simulink model "VehDyn14DOF"  (R2025a)
settings: Solver=VariableStepAuto  StartTime=0.0  StopTime=inf  FixedStep=0.001  RelTol=1e-3
model workspace (MAT data in the model file):
  ssEnable = Simulink.Parameter
  ssEnable.Value = 0
  ssEnable.Complexity = 'real'
  ssEnable.Dimensions = [1 1]
  ssEnable.DataType = 'boolean'
  xdot_r = Simulink.Parameter
  xdot_r.Value = 2.7778
  xdot_r.Complexity = 'real'
  xdot_r.Dimensions = [1 1]
  xdot_r.DataType = 'auto'
values from neighbouring files (symbols this model uses):
  AccPwrbp = 0.0 3.0779560993538198    [vehDyn14DOF.sldd]
  AccSpdbp = 256.49641719585139 641.24104298962845    [vehDyn14DOF.sldd]
  Downshift_Speeds = 9.5625 12.9375 16.3125 19.6875 23.0625 26.4375 29.8125 33.1875 36.5625 39.9375 43.3125 46.687499999999986 47.8125 51.187499999999986 54.562499999999986 57.9375 59.0625 62.4375 65.8125 69.1875 68.90625 72.84375 76.78125 80.71875 78.75 83.25 87.75 92.25    [vehDyn14DOF.sldd]
  EngRevLim = 7000.0    [vehDyn14DOF.sldd]
  F0z = 2886.0 2907.0    [vehDyn14DOF.sldd]
  Pedal_Positions = 0.1 0.4 0.5 0.9    [vehDyn14DOF.sldd]
  Trans = 0.01    [vehDyn14DOF.sldd]
  Upshift_Speeds = 12.9375 16.3125 19.6875 33.0 26.4375 29.8125 33.1875 52.5 39.9375 43.3125 46.687499999999986 77.25 51.187499999999986 54.562499999999986 57.9375 100.5 62.4375 65.8125 69.1875 138.75 72.84375 76.78125 80.71875 161.875 83.25 87.75 92.25 185.0    [vehDyn14DOF.sldd]
  VEH = 1575.0    [vehDyn14DOF.sldd]
undefined symbols (not defined in the file or in its folder): AccelCmd, CurvGradRef, CurvRef, DecelCmd, DiscIntNeverNeededParam, egoVehDyn, EnblAccelCmd, EnblDecelCmd, EnblSteerCmd, GearCmd, Gnd, Iz, lambda_mux, lambda_muy, lf, LngRef, lr, LtrRef, m, max_dc, maxSteer, PhiRef, SteerCmd, steeringGain, SteerZero, Wind, XRef, YRef, Z
libraries: simulink x14, autolibutils x13, autolibsharedcoupling x11, vehdynlibtire x10, vehdynlibsuspension x8, sharedtransform x5, autolibshareddiff x5, shared6dof x2, slpidlib x1, autolibtranscontrolscommon x1, vehdynlibdriver x1, autolibshared x1
(part 1 of 10)
CloseFcn:
  | Simulink.data.dictionary.closeAll('vehDyn14DOF.sldd', '-discard')
settings Model: DataDictionary=vehDyn14DOF.sldd  Creator=The MathWorks, Inc.  LastModifiedBy=sdussani
settings SolverCC: MaxZcPerStep=1.0
settings DataIOCC: InitialState=refModelOP  SignalLogging=off
settings OptimizationCC: ReuseModelBlockBuffer=off  ZeroExternalMemoryAtStartup=off  ZeroInternalMemoryAtStartup=off
settings DebuggingCC: UnconnectedInputMsg=warning  UnconnectedOutputMsg=warning  UnconnectedLineMsg=warning  SubsystemReferenceDiagnosticForUnitTest=warning
settings ModelReferenceCC: EnableRefExpFcnMdlSchedulingChecks=on
settings RTWCC: GenerateReport=on  LaunchReport=on  TargetLang=C++  GPUComputeCapability=3.5  DLArmComputeVersion=19.05
settings GRTTargetCC: TargetLangStandard=C++03 (ISO)  MatFileLogging=off  CodeInterfacePackaging=C++ class

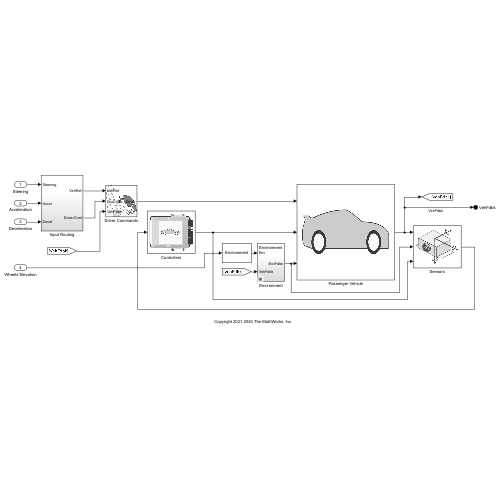
[thumbnail: Simulink's stored preview of the top-level diagram]
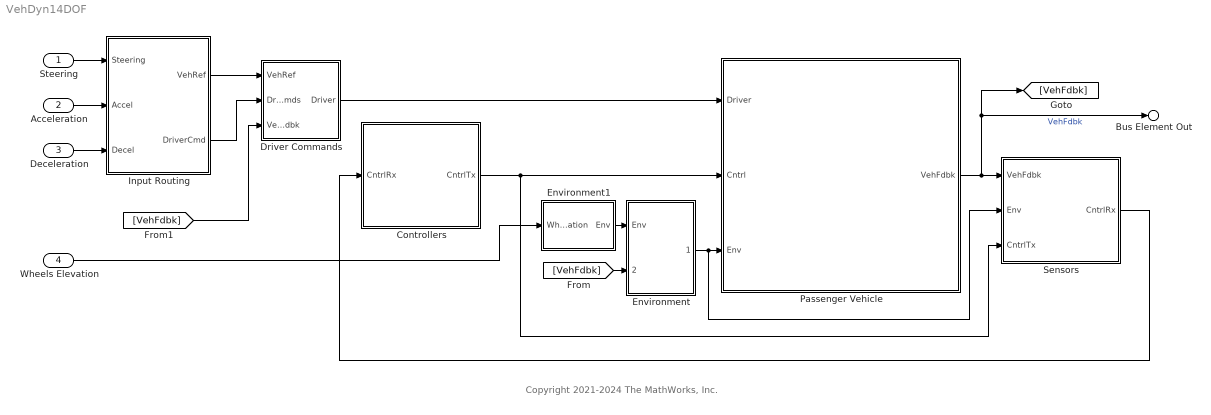
== system VehDyn14DOF ==
  note: Copyright 2021-2024 The MathWorks, Inc.
  Steering : Inport
  Acceleration : Inport  Port=2
  Deceleration : Inport  Port=3
  Wheels Elevation : Inport  Port=4
  Controllers : Subsystem
      mask Display: image('$imagefile'); % Use "Edit Image" on toolstrip to change.
  Driver Commands : Subsystem  VariantControl=0
      mask Display: image('driverlatlong.png');
  Environment : Subsystem  Variant=on  VariantControlMode=label  VariantControl=Choice  LabelModeActiveChoice=Choice
  Environment1 : Subsystem
      mask Display: disp('Environment')
  Input Routing : Subsystem  VariantControl=0
  Passenger Vehicle : Subsystem
      mask Display: image('$imagefile'); % Use "Edit Image" on toolstrip to change.
  Sensors : Subsystem
      mask Display: image('sensorimu.png'); % Use "Edit Image" on toolstrip to change.
  Bus Element Out : Outport  PortName=VehFdbk
  wires:
  Passenger Vehicle/1(VehFdbk) -> Bus Element Out/1, [VehFdbk], Sensors/1(VehFdbk)  "VehFdbk"
  Sensors/1(CntrlRx) -> Controllers/1(CntrlRx)
  Controllers/1(CntrlTx) -> Passenger Vehicle/2(Cntrl), Sensors/3(CntrlTx)
  Driver Commands/1(Driver) -> Passenger Vehicle/1(Driver)
  Input Routing/1(VehRef) -> Driver Commands/1(VehRef)
  Input Routing/2(DriverCmd) -> Driver Commands/2(DrvCmds)
  Environment1/1(Env) -> Environment/1(Env)
  [VehFdbk] -> Environment/2(VehFdbk)
  Environment/1(EnvFdbk) -> Sensors/2(Env), Passenger Vehicle/3(Env)
  [VehFdbk] -> Driver Commands/3(VehFdbk)
  Acceleration/1 -> Input Routing/2(Accel)
  Steering/1 -> Input Routing/1(Steering)
  Deceleration/1 -> Input Routing/3(Decel)
  Wheels Elevation/1 -> Environment1/1(Wheels Elevation)

== system VehDyn14DOF/Controllers ==
  CntrlRx : Inport
  Active Differential Control : Subsystem  Variant=on  VariantControlMode=label  LabelModeActiveChoice=0
  Brake Pressure Control : Subsystem  Variant=on  VariantControlMode=label  LabelModeActiveChoice=0
  Bus Creator : BusCreator  Inputs=1
  Bus Creator1 : BusCreator  Inputs=1
  Bus Creator2 : BusCreator  Inputs=2
  Bus Creator3 : BusCreator  Inputs=4
  Bus Creator4 : BusCreator  Inputs=1
  Bus Selector : BusSelector  OutputSignals=Driver.DecelFdbk,Wheels.Omega,IMU.Acc
  Bus Selector1 : BusSelector  OutputSignals=Driver.AccFdbk,Driver.DecelFdbk,Driver.GearFdbk,Engine.EngSpd,Wheels.Omega
  Bus Selector2 : BusSelector  OutputSignals=Driver.AccFdbk,Engine.EngSpd
  Bus Selector3 : BusSelector  OutputSignals=Driver.AccFdbk,Driver.DecelFdbk,Driver.SteerFdbk,Driver.GearFdbk,Wheels.Omega,IMU.Acc,IMU.pqr
  ECU : Subsystem  SystemSampleTime=.01
  Ground : Ground
  Transmission Controller : Subsystem  Variant=on  VariantControlMode=label  VariantControl=Variant1  LabelModeActiveChoice=3
  CntrlTx : Outport  VectorParamsAs1DForOutWhenUnconnected=off
  wires:
  Bus Selector2/1 -> ECU/2(<Accel>)  "<AccFdbk>"
  Bus Creator/1 -> Bus Creator3/1  "ECU"
  Bus Creator1/1 -> Bus Creator3/2  "Transmission"
  Bus Creator3/1 -> CntrlTx/1  "CntrlTx"
  Bus Creator4/1 -> Bus Creator3/4  "Diff"
  Active Differential Control/1(DiffPrsCmd) -> Bus Creator4/1  "DiffPrsCmd"
  Active Differential Control/2(TrqCmd) -> [DiffTrqCmd]
  ECU/1(EngTrqCmd) -> Bus Creator/1  "EngTrqCmd"
  Transmission Controller/1(" Gear") -> Bus Creator1/1  "GearCmd"
  [DiffTrqCmd] -> ECU/1(DiffTrqCmd)  "DiffTrqCmd"
  Ground/1 -> Transmission Controller/7(UpReq), Transmission Controller/8(DownReq)
  Bus Selector2/2 -> ECU/3(EngSpd)  "<EngSpd>"
  Bus Selector1/5 -> Transmission Controller/5(Omega)  "<Omega>"
  Bus Selector1/2 -> Transmission Controller/2(BrkCmd)  "<DecelFdbk>"
  Bus Selector1/3 -> Transmission Controller/3(GearReq)  "<GearFdbk>"
  Bus Selector1/4 -> Transmission Controller/4(EngSpd)  "<EngSpd>"
  Bus Selector1/1 -> Transmission Controller/1(Accel)  "<AccFdbk>"
  Bus Selector3/1 -> Active Differential Control/1(Accel)  "<AccFdbk>"
  Bus Selector3/2 -> Active Differential Control/2(BrkCmd)  "<DecelFdbk>"
  Bus Selector3/3 -> Active Differential Control/3(Steer)  "<SteerFdbk>"
  Bus Selector3/4 -> Active Differential Control/4(GearFdbk)  "<GearFdbk>"
  Bus Selector3/5 -> Active Differential Control/5(Omega)  "<Omega>"
  Bus Selector3/6 -> Active Differential Control/6(axayaz)  "<Acc>"
  Bus Selector3/7 -> Active Differential Control/7(pqr)  "<pqr>"
  Bus Selector/1 -> Brake Pressure Control/1(DecelFdbk)  "<DecelFdbk>"
  CntrlRx/1 -> Bus Selector/1, Bus Selector3/1, Bus Selector1/1, Bus Selector2/1
  Bus Selector/2 -> Brake Pressure Control/2(Omega)  "<Omega>"
  Bus Selector/3 -> Brake Pressure Control/3(Accel)  "<Acc>"
  Brake Pressure Control/1(BrkPrsCmd) -> Bus Creator2/1  "BrkPrsCmd"
  Bus Creator2/1 -> Bus Creator3/3  "Brake"
  Brake Pressure Control/2(ABSFlag) -> Bus Creator2/2, [ABSFlag]  "ABSFlag"
  [ABSFlag] -> Transmission Controller/6(ABSFlag)
  [ABSFlag] -> ECU/4(ABSFlag)

== system VehDyn14DOF/Driver Commands ==
  VehRef : Inport  OutDataTypeStr=Bus: BusVehRef
  DrvCmds : Inport  Port=2  OutDataTypeStr=Bus: BusDrvCmds
  VehFdbk : Inport  Port=3
  Bus Creator1 : BusCreator  Inputs=5
  Bus Selector : BusSelector  OutputSignals=Body.BdyFrm.Cg.Vel.xdot,Body.InertFrm.Geom.Disp.X,Body.InertFrm.Geom.Disp.Y,Body.InertFrm.Cg.Ang.psi,Body.BdyFrm.Cg.AngVel.r
  Bus Selector1 : BusSelector  OutputSignals=EnblSteerCmd,SteerCmd,SteerHld,SteerZero,EnblAccelCmd,AccelCmd,AccelHld,AccelZero,EnblDecelCmd,DecelCmd,DecelHld,DecelZero
  Bus Selector2 : BusSelector  OutputSignals=LngRef,XRef,YRef,PhiRef,CurvRef
  Dead Zone : DeadZone  LowerValue=-.5  UpperValue=.5  ZeroCross=off
  Gain : Gain  Gain=18*maxSteer
  Ground : Ground
  Ground1 : Ground
  Linear Predictive Driver : vehdynlibdriver/Predictive Driver  extAccelOvr=on  extDecelOvr=on  extAccelHld=on  extDecelHld=on  extAccelZero=on  extDecelZero=on  extSteerOvr=on  extSteerHld=on  extSteerZero=on  cntrlType=Predictive  cntrlTypeLat=Stanley  shftType=Reverse, Neutral, Drive  coordMode=SAE J670 (Z-down)  refType=Reference pose  velUnits=m/s  angUnits=rad  gearOut=on  steerOut=on  Kp=3  Ki=1  Kff=1  Kg=0  VehVelVec=[0 100]  KffVec=[.1 .1]  KpVec=[10 10]  KiVec=[5 5]  KgVec=[0 0]  vnom=5  Kaw=1  tauerr=.075  tau=.15  L=6  Kpt=20000  aR=200  bR=2.5  cR=.5  g=9.81  vecPose=off  dynamMode=on  PositionGainF=2.5  PositionGainR=2.5  YawRateGain=.2  DelayGain=.2  enableDrift=off  BetaRef=20*pi/180  KpBeta=1  KpDrift=2  KdDrift=1  KpPsi=6  KOmega=30  tOmega=1  a=VEH.FrontAxlePositionfromCG  b=VEH.RearAxlePositionfromCG  m=VEH.Mass  Cy_f=5000  Cy_r=7000  I=VEH.YawMomentInertia  Ksteer=18  theta=40*pi/180  Idl=1  Re=.3  lambda_mu=1  GearInit=1  tShift=.1  pdlVec=[0.1 0.4 0.5 0.9]  upShftTbl=[-1 12.9375 26.4375 39.9375 51.18749999999999 62.4375 72.84375 83.25;-1 16.3125 29.8125 43.3125 54.5624 65.8125 76.78125 87.75;-1 19.6875 33.1875 46.68749999999999 57.9375 69.1875 80.71875 92.25;-1 33 52.5 77.25 100.5 138.75 161.875 185]  dwnShftTbl=[-1 12.9375 26.4375 39.9375 51.18749999999999 62.4375 72.84375 83.25;-1 16.3125 29.8125 43.3125 54.5624 65.8125 76.78125 87.75;-1 19.6875 33.1875 46.68749999999999 57.9375 69.1875 80.71875 92.25;-1 33 52.5 77.25 100.5 138.75 161.875 185]  tClutch=.5  tRev=.5  tPark=120  UpGearVec="[0  1  2  3  4  5  6  7]"  DownGearVec="[1  2  3  4  5  6  7  8]"  aMode=2
  Mux : Mux  Inputs=3
  Steady State : Subsystem  VariantControl=Choice
  Terminator : Terminator
  Driver : Outport  VectorParamsAs1DForOutWhenUnconnected=off
  wires:
  Bus Creator1/1 -> Driver/1
  Bus Selector2/1 -> Linear Predictive Driver/1  "<LngRef>"
  VehFdbk/1 -> Bus Selector/1
  Bus Selector/2 -> Linear Predictive Driver/20  "<X>"
  Linear Predictive Driver/4 -> Bus Creator1/3  "decel_cmd"
  Linear Predictive Driver/2 -> Bus Creator1/1  "steer_cmd"
  Ground/1 -> Linear Predictive Driver/17
  Linear Predictive Driver/1 -> Terminator/1
  Linear Predictive Driver/3 -> Bus Creator1/2  "accel_cmd"
  Bus Selector/4 -> Linear Predictive Driver/22  "<psi>"
  Bus Selector/5 -> Linear Predictive Driver/23  "<r>"
  Bus Selector/1 -> Dead Zone/1  "<xdot>"
  Linear Predictive Driver/5 -> Bus Creator1/4  "gear_cmd"
  Bus Selector/3 -> Linear Predictive Driver/21  "<Y>"
  Dead Zone/1 -> Linear Predictive Driver/19
  Ground1/1 -> Mux/3
  Mux/1 -> Bus Creator1/5  "Ref"
  DrvCmds/1 -> Steady State/2(DrvCmds)
  Bus Selector1/1 -> Linear Predictive Driver/5  "<EnblSteerCmd>"
  Bus Selector1/2 -> Gain/1  "<SteerCmd>"
  Bus Selector1/3 -> Linear Predictive Driver/7  "<SteerHld>"
  Bus Selector1/4 -> Linear Predictive Driver/8  "<SteerZero>"
  Bus Selector1/5 -> Linear Predictive Driver/9  "<EnblAccelCmd>"
  Bus Selector1/6 -> Linear Predictive Driver/10  "<AccelCmd>"
  Bus Selector1/7 -> Linear Predictive Driver/11  "<AccelHld>"
  Bus Selector1/8 -> Linear Predictive Driver/12  "<AccelZero>"
  Bus Selector1/9 -> Linear Predictive Driver/13  "<EnblDecelCmd>"
  Bus Selector1/10 -> Linear Predictive Driver/14  "<DecelCmd>"
  Bus Selector1/11 -> Linear Predictive Driver/15  "<DecelHld>"
  Bus Selector1/12 -> Linear Predictive Driver/16  "<DecelZero>"
  VehRef/1 -> Steady State/1(VehRef)
  Bus Selector2/2 -> Mux/1, Linear Predictive Driver/2  "<XRef>"
  Bus Selector2/3 -> Mux/2, Linear Predictive Driver/3  "<YRef>"
  Bus Selector2/4 -> Linear Predictive Driver/4  "<PhiRef>"
  Bus Selector2/5 -> Linear Predictive Driver/18  "<CurvRef>"
  Steady State/1(Ref) -> Bus Selector2/1
  Steady State/2(Cmds) -> Bus Selector1/1
  Gain/1 -> Linear Predictive Driver/6

== system VehDyn14DOF/Environment ==
  Env : Inport
  VehFdbk : Inport  Port=2
  Environment : Subsystem  VariantControl=Choice
  EnvFdbk : Outport

== system VehDyn14DOF/Environment1 ==
  Wheels Elevation : Inport
  Bus Assignment : BusAssignment  AssignedSignals=Wind,Gnd
  Constant1 : Constant  Value=0  OutDataTypeStr=Bus: BusEnv  SampleTime=-1
  Constant3 : Constant  Value=0  SampleTime=-1
  Constant4 : Constant  Value=0  SampleTime=-1
  Constant5 : Constant  Value=0  SampleTime=-1
  Friction : Constant  Value=ones(4,1).*1  SampleTime=-1
  Ground Feedback : Subsystem  VariantControl=0
  Vector Concatenate : Concatenate  NumInputs=3
  Env : Outport  VectorParamsAs1DForOutWhenUnconnected=off
  wires:
  Constant1/1 -> Bus Assignment/1
  Bus Assignment/1 -> Env/1
  Ground Feedback/1(Ground) -> Bus Assignment/3  "Gnd"
  Vector Concatenate/1 -> Bus Assignment/2  "Wind"
  Friction/1 -> Ground Feedback/1(Friction)
  Constant4/1 -> Vector Concatenate/2  "Y"
  Constant3/1 -> Vector Concatenate/1  "X"
  Constant5/1 -> Vector Concatenate/3  "Z"
  Wheels Elevation/1 -> Ground Feedback/2(Wheels Elevation)

== system VehDyn14DOF/Input Routing ==
  Steering : Inport  Unit=rad  PortDimensions=1
  Accel : Inport  Port=2  Unit=m/s^2  PortDimensions=1
  Decel : Inport  Port=3  Unit=m/s^2  PortDimensions=1
  Bus Assignment : BusAssignment  AssignedSignals=EnblDecelCmd,EnblAccelCmd,EnblSteerCmd,SteerCmd,AccelCmd,DecelCmd,GearCmd
  Constant : Constant  Value=int8(1)  SampleTime=-1
  Constant1 : Constant  Value=0  OutDataTypeStr=Bus: BusDrvCmds  SampleTime=-1
  Constant2 : Constant  Value=true  SampleTime=-1
  FrontWheelScaling : Gain  Gain=steeringGain
  Product : Product
  Product1 : Product
  Product2 : Product
  Ramp : simulink/Sources/Ramp  slope=10  start=0  InitialOutput=0
  Saturation : Saturate  UpperLimit=1  LowerLimit=0
  Saturation1 : Saturate  UpperLimit=4  LowerLimit=0
  Saturation2 : Saturate  UpperLimit=4  LowerLimit=max_dc
  Signal Specification : SignalSpecification  Unit=one
  Signal Specification1 : SignalSpecification  Unit=1
  Signal Specification2 : SignalSpecification  Unit=1
  Signal Specification3 : SignalSpecification  Unit=1
  Vehicle Reference : Subsystem
  m/s^2 to torque request : Gain  Gain=1/4
  m/s^2 to torque request1 : Gain  Gain=1/4
  VehRef : Outport
  DriverCmd : Outport  Port=2
  wires:
  Constant2/1 -> Bus Assignment/2, Bus Assignment/3, Bus Assignment/4
  Constant1/1 -> Bus Assignment/1
  Bus Assignment/1 -> DriverCmd/1
  Vehicle Reference/1(VehRef) -> VehRef/1
  Saturation1/1 -> Product1/2
  Saturation2/1 -> Product2/2
  Product2/1 -> m/s^2 to torque request1/1
  Product1/1 -> m/s^2 to torque request/1
  Saturation/1 -> Product/1, Product1/1, Product2/1
  Product/1 -> FrontWheelScaling/1
  Ramp/1 -> Saturation/1
  Signal Specification/1 -> Bus Assignment/5  "SteerCmd"
  m/s^2 to torque request/1 -> Signal Specification1/1
  FrontWheelScaling/1 -> Signal Specification/1
  Signal Specification1/1 -> Bus Assignment/6  "AccelCmd"
  Signal Specification3/1 -> Bus Assignment/8  "GearCmd"
  Signal Specification2/1 -> Bus Assignment/7  "DecelCmd"
  Constant/1 -> Signal Specification3/1  "PRNDL"
  Accel/1 -> Saturation1/1
  Decel/1 -> Saturation2/1
  m/s^2 to torque request1/1 -> Signal Specification2/1
  Steering/1 -> Product/2

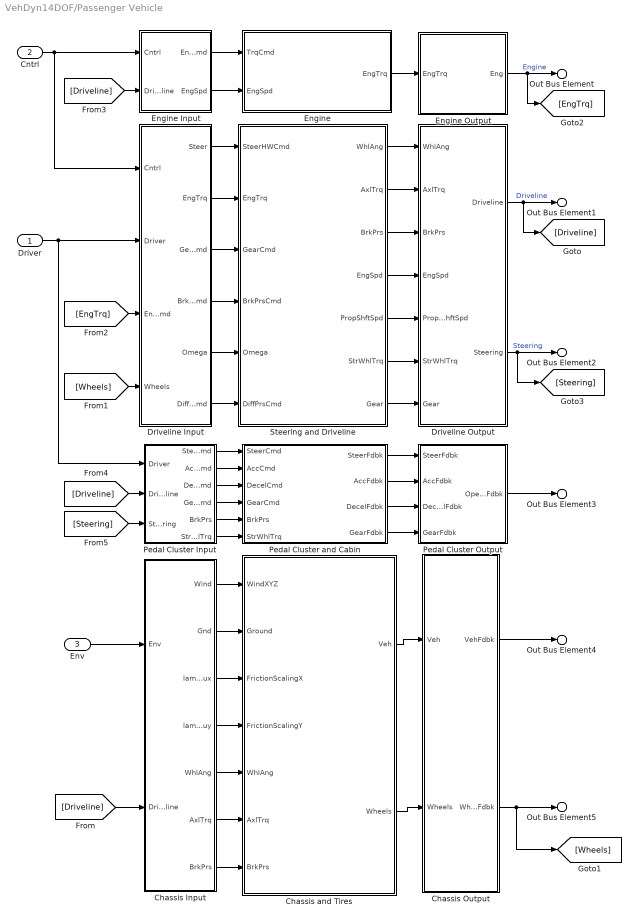
== system VehDyn14DOF/Passenger Vehicle ==
  Driver : Inport
  Cntrl : Inport  Port=2
  Env : Inport  Port=3
  Chassis Input : Subsystem
  Chassis Output : Subsystem
  Chassis and Tires : Subsystem
  Driveline Input : Subsystem
  Driveline Output : Subsystem
  Engine : Subsystem
  Engine Input : Subsystem
  Engine Output : Subsystem
  Pedal Cluster Input : Subsystem
  Pedal Cluster Output : Subsystem
  Pedal Cluster and Cabin : Subsystem
  Steering and Driveline : Subsystem
  Out Bus Element : Outport  PortName=VehFdbk  Element=Engine
  Out Bus Element1 : Outport  PortName=VehFdbk  Element=Driveline
  Out Bus Element2 : Outport  PortName=VehFdbk  Element=Steering
  Out Bus Element3 : Outport  PortName=VehFdbk  Element=Driver
  Out Bus Element4 : Outport  PortName=VehFdbk  Element=Body
  Out Bus Element5 : Outport  PortName=VehFdbk  Element=Wheels
  wires:
  Env/1 -> Chassis Input/1(Env)
  Driveline Output/1(Driveline) -> Out Bus Element1/1, [Driveline]  "Driveline"
  Steering and Driveline/1(WhlAng) -> Driveline Output/1(WhlAng)
  Steering and Driveline/2(AxlTrq) -> Driveline Output/2(AxlTrq)
  Steering and Driveline/3(BrkPrs) -> Driveline Output/3(BrkPrs)
  Steering and Driveline/4(EngSpd) -> Driveline Output/4(EngSpd)
  Steering and Driveline/5(PropShftSpd) -> Driveline Output/5(PropShftSpd)
  Driver/1 -> Pedal Cluster Input/1(Driver), Driveline Input/2(Driver)
  Cntrl/1 -> Engine Input/1(Cntrl), Driveline Input/1(Cntrl)
  Driveline Input/1(Steer) -> Steering and Driveline/1(SteerHWCmd)
  Driveline Input/3(GearCmd) -> Steering and Driveline/3(GearCmd)
  Driveline Input/4(BrkPrsCmd) -> Steering and Driveline/4(BrkPrsCmd)
  Driveline Input/5(Omega) -> Steering and Driveline/5(Omega)
  Engine/1(EngTrq) -> Engine Output/1("EngTrq ")
  Driveline Input/2(EngTrq) -> Steering and Driveline/2(EngTrq)
  Engine Input/1(EngTrqCmd) -> Engine/1(TrqCmd)
  Engine Input/2(EngSpd) -> Engine/2(EngSpd)
  Engine Output/1(Eng) -> Out Bus Element/1, [EngTrq]  "Engine"
  [Driveline] -> Chassis Input/2(Driveline)
  [Wheels] -> Driveline Input/4(Wheels)
  [EngTrq] -> Driveline Input/3(EngTrqCmd)
  [Driveline] -> Engine Input/2(Driveline)
  Driveline Input/6(DiffPrsCmd) -> Steering and Driveline/6(DiffPrsCmd)
  Steering and Driveline/6(StrWhlTrq) -> Driveline Output/6(StrWhlTrq)
  Driveline Output/2(Steering) -> Out Bus Element2/1, [Steering]  "Steering"
  Pedal Cluster Output/1(OperatorFdbk) -> Out Bus Element3/1
  Pedal Cluster and Cabin/1(SteerFdbk) -> Pedal Cluster Output/1(SteerFdbk)
  Pedal Cluster and Cabin/2(AccFdbk) -> Pedal Cluster Output/2(AccFdbk)
  Pedal Cluster and Cabin/3(DecelFdbk) -> Pedal Cluster Output/3(DecelFdbk)
  Pedal Cluster and Cabin/4(GearFdbk) -> Pedal Cluster Output/4(GearFdbk)
  Pedal Cluster Input/4(GearCmd) -> Pedal Cluster and Cabin/4(GearCmd)
  Pedal Cluster Input/3(DecelCmd) -> Pedal Cluster and Cabin/3(DecelCmd)
  Pedal Cluster Input/2(AccelCmd) -> Pedal Cluster and Cabin/2(AccCmd)
  Pedal Cluster Input/1(SteerCmd) -> Pedal Cluster and Cabin/1(SteerCmd)
  [Driveline] -> Pedal Cluster Input/2(Driveline)
  Pedal Cluster Input/5(BrkPrs) -> Pedal Cluster and Cabin/5(BrkPrs)
  [Steering] -> Pedal Cluster Input/3(Steering)
  Pedal Cluster Input/6(StrWhlTrq) -> Pedal Cluster and Cabin/6(StrWhlTrq)
  Chassis and Tires/2(Wheels) -> Chassis Output/2(Wheels)
  Chassis and Tires/1(Veh) -> Chassis Output/1(Veh)
  Chassis Output/2(WheelsFdbk) -> [Wheels], Out Bus Element5/1
  Chassis Output/1(VehFdbk) -> Out Bus Element4/1
  Steering and Driveline/7(Gear) -> Driveline Output/7(Gear)
  Chassis Input/1(Wind) -> Chassis and Tires/1(WindXYZ)
  Chassis Input/2(Gnd) -> Chassis and Tires/2(Ground)
  Chassis Input/3(lambda_mux) -> Chassis and Tires/3(FrictionScalingX)
  Chassis Input/5(WhlAng) -> Chassis and Tires/5(WhlAng)
  Chassis Input/6(AxlTrq) -> Chassis and Tires/6(AxlTrq)
  Chassis Input/7(BrkPrs) -> Chassis and Tires/7(BrkPrs)
  Chassis Input/4(lambda_muy) -> Chassis and Tires/4(FrictionScalingY)

== system VehDyn14DOF/Sensors ==
  VehFdbk : Inport
  Env : Inport  Port=2
  CntrlTx : Inport  Port=3
  Bus Creator1 : BusCreator  Inputs=2
  Bus Selector : BusSelector  OutputSignals=Body.BdyFrm.Cg.Acc.ax,Body.BdyFrm.Cg.Acc.ay,Body.BdyFrm.Cg.Acc.az  OutputAsBus=on
  Bus Selector1 : BusSelector  OutputSignals=Body.BdyFrm.Cg.AngVel.p,Body.BdyFrm.Cg.AngVel.q,Body.BdyFrm.Cg.AngVel.r  OutputAsBus=on
  Bus Selector2 : BusSelector  OutputSignals=Body.BdyFrm.Cg.AngAcc.pdot,Body.BdyFrm.Cg.AngAcc.qdot,Body.BdyFrm.Cg.AngAcc.rdot  OutputAsBus=on
  Bus Selector3 : BusSelector  OutputSignals=Driver  OutputAsBus=on
  Bus Selector4 : BusSelector  OutputSignals=Engine.EngTrq,Driveline.EngSpd  OutputAsBus=on
  Bus Selector5 : BusSelector  OutputSignals=Driveline.BrkPrs,Wheels.TireFrame.Kappa,Wheels.TireFrame.Alpha,Wheels.TireFrame.Omega  OutputAsBus=on
  Bus Selector6 : BusSelector  OutputSignals=Driveline.PropShftSpd,Driveline.AxlTrq  OutputAsBus=on
  Bus to Vector : BusToVector
  Bus to Vector1 : BusToVector
  Bus to Vector2 : BusToVector
  Constant : Constant  Value=[0,0,0]
  Constant1 : Constant  Value=[0,0,9.81]
  Terminator : Terminator
  Three-axis Inertial Measurement Unit : vehdynlibsens/Three-axis Inertial Measurement Unit  units=Metric (MKS)  imu=[0 0 0]  i_Ts=0  dtype_a=off  w_a=190  z_a=0.707  a_sf_cc=[1 0 0; 0 1 0; 0 0 1]  a_bias=[0 0 0]  a_sat="[-inf  -inf  -inf  inf inf inf]"  dtype_g=off  w_g=190  z_g=0.707  g_sf_cc=[1 0 0; 0 1 0; 0 0 1]  g_bias=[0 0 0]  g_sens=[0 0 0]  g_sat="[-inf  -inf  -inf  inf inf inf]"  i_rand=on  i_seeds=[23093 23094 23095 23096 23097 23098]  i_pow=[0.001 0.001 0.001 0.0001 0.0001 0.0001]  aMode=2
  Unit Conversion : UnitConversion
  Out Bus Element : Outport  PortName=CntrlRx  Element=Driver
  Out Bus Element1 : Outport  PortName=CntrlRx  Element=Engine
  Out Bus Element2 : Outport  PortName=CntrlRx  Element=Trans
  Out Bus Element3 : Outport  PortName=CntrlRx  Element=Wheels
  Out Bus Element4 : Outport  PortName=CntrlRx  Element=IMU
  Out Bus Element5 : Outport  PortName=CntrlRx  Element=Env
  wires:
  VehFdbk/1 -> Bus Selector/1, Bus Selector2/1, Bus Selector1/1, Bus Selector6/1, Bus Selector3/1, Bus Selector4/1, Bus Selector5/1  "VehFdbk"
  Bus Creator1/1 -> Out Bus Element4/1
  Three-axis Inertial Measurement Unit/1 -> Bus Creator1/1  "Acc"
  Three-axis Inertial Measurement Unit/2 -> Bus Creator1/2  "pqr"
  Bus Selector/1 -> Bus to Vector/1
  Bus to Vector/1 -> Unit Conversion/1
  Bus Selector1/1 -> Bus to Vector1/1
  Bus to Vector1/1 -> Three-axis Inertial Measurement Unit/2
  Env/1 -> Out Bus Element5/1
  Bus Selector2/1 -> Bus to Vector2/1
  Bus to Vector2/1 -> Three-axis Inertial Measurement Unit/3
  Constant/1 -> Three-axis Inertial Measurement Unit/4
  Constant1/1 -> Three-axis Inertial Measurement Unit/5
  Unit Conversion/1 -> Three-axis Inertial Measurement Unit/1
  CntrlTx/1 -> Terminator/1
  Bus Selector3/1 -> Out Bus Element/1
  Bus Selector4/1 -> Out Bus Element1/1
  Bus Selector5/1 -> Out Bus Element3/1
  Bus Selector6/1 -> Out Bus Element2/1

== system VehDyn14DOF/Controllers/Active Differential Control ==
  note: 1) Add Subsystem or Model blocks as valid variant choices.
      | 2) You cannot connect blocks at this level. At simulation, connectivity is automatically
      | determined, based on the active variant and port name matching.
  Accel : Inport
  BrkCmd : Inport  Port=2
  Steer : Inport  Port=3
  GearFdbk : Inport  Port=4
  Omega : Inport  Port=5  Unit=rad/s
  axayaz : Inport  Port=6
  pqr : Inport  Port=7
  No Control : Subsystem  VariantControl=0
  Rear Diff Controller : Subsystem  TreatAsAtomicUnit=on  SystemSampleTime=.01  VariantControl=1
  DiffPrsCmd : Outport  VectorParamsAs1DForOutWhenUnconnected=off
  TrqCmd : Outport  Port=2  VectorParamsAs1DForOutWhenUnconnected=off

== system VehDyn14DOF/Controllers/Brake Pressure Control ==
  note: 1) Add Subsystem or Model blocks as valid variant choices.
      | 2) You cannot connect blocks at this level. At simulation, connectivity is automatically
      | determined, based on the active variant and port name matching.
  DecelFdbk : Inport
  Omega : Inport  Port=2
  Accel : Inport  Port=3
  Bang Bang ABS : Subsystem  VariantControl=1
  Five-State ABS : Subsystem  VariantControl=2
  Open Loop : Subsystem  VariantControl=0
  BrkPrsCmd : Outport  VectorParamsAs1DForOutWhenUnconnected=off
  ABSFlag : Outport  Port=2  VectorParamsAs1DForOutWhenUnconnected=off

== system VehDyn14DOF/Controllers/ECU ==
  DiffTrqCmd : Inport
  <Accel> : Inport  Port=2
  EngSpd : Inport  Port=3
  ABSFlag : Inport  Port=4
  First Order Hold : FirstOrderHold  ErrorTolerance=100
  Torque Cmd : Subsystem  TreatAsAtomicUnit=on  SystemSampleTime=.01
  EngTrqCmd : Outport  VectorParamsAs1DForOutWhenUnconnected=off
  wires:
  First Order Hold/1 -> EngTrqCmd/1
  DiffTrqCmd/1 -> Torque Cmd/1(DiffTrqCmd)
  <Accel>/1 -> Torque Cmd/2(<Accel>)
  EngSpd/1 -> Torque Cmd/3(EngSpd)
  Torque Cmd/1(EngTrqCmd) -> First Order Hold/1
  ABSFlag/1 -> Torque Cmd/4(ABSFlag)

== system VehDyn14DOF/Controllers/Transmission Controller ==
  Accel : Inport
  BrkCmd : Inport  Port=2
  GearReq : Inport  Port=3
  EngSpd : Inport  Port=4
  Omega : Inport  Port=5  Unit=rad/s  PortDimensions=4
  ABSFlag : Inport  Port=6
  UpReq : Inport  Port=7
  DownReq : Inport  Port=8  Unit=rad/s
  Driver - No Clutch : Subsystem  VariantControl=1
  PRNDL Controller : Subsystem  VariantControl=3
  Paddles : Subsystem  VariantControl=2
  Transmission Controller : Subsystem  VariantControl=0
  " Gear" : Outport  VectorParamsAs1DForOutWhenUnconnected=off

== system VehDyn14DOF/Driver Commands/Steady State ==
  VehRef : Inport
  DrvCmds : Inport  Port=2
  Bus Assignment : BusAssignment  AssignedSignals=LngRef
  Bus Assignment1 : BusAssignment  AssignedSignals=EnblSteerCmd,SteerZero,EnblAccelCmd,EnblDecelCmd
  Constant2 : Constant  Value=true
  Constant3 : Constant  Value=false
  EnableSS : Constant  Value=ssEnable
  Ramp : simulink/Sources/Ramp  slope=10  start=1  InitialOutput=0
  Saturation : Saturate  UpperLimit=xdot_r  LowerLimit=-inf
  Signal Specification : SignalSpecification  Unit=m/s
  Switch : Switch  Criteria=u2 > Threshold  SaturateOnIntegerOverflow=off  InputSameDT=off
  Switch1 : Switch  Criteria=u2 > Threshold  SaturateOnIntegerOverflow=off  InputSameDT=off
  Ref : Outport  OutDataTypeStr=Bus: BusVehRef
  Cmds : Outport  Port=2  OutDataTypeStr=Bus: BusDrvCmds
  wires:
  Bus Assignment/1 -> Switch/1
  VehRef/1 -> Switch/3, Bus Assignment/1
  Bus Assignment1/1 -> Switch1/1
  DrvCmds/1 -> Bus Assignment1/1, Switch1/3
  Ramp/1 -> Saturation/1
  Saturation/1 -> Signal Specification/1
  Constant2/1 -> Bus Assignment1/2, Bus Assignment1/3
  Constant3/1 -> Bus Assignment1/4, Bus Assignment1/5
  Switch/1 -> Ref/1
  Switch1/1 -> Cmds/1
  EnableSS/1 -> Switch/2, Switch1/2
  Signal Specification/1 -> Bus Assignment/2

== system VehDyn14DOF/Environment/Environment ==
  Env : Inport
  VehFdbk : Inport  Port=2
  Bus Assignment : BusAssignment  AssignedSignals=Gnd.lambda_mux,Gnd.lambda_muy
  Constant : Constant  Value=ones(4,1)
  Terminator : Terminator
  EnvFdbk : Outport
  wires:
  Env/1 -> Bus Assignment/1
  Constant/1 -> Bus Assignment/3, Bus Assignment/2
  Bus Assignment/1 -> EnvFdbk/1
  VehFdbk/1 -> Terminator/1

== system VehDyn14DOF/Environment1/Ground Feedback ==
  Friction : Inport
  Wheels Elevation : Inport  Port=2
  Bus Assignment : BusAssignment  AssignedSignals=Z,lambda_mux,lambda_muy
  Constant4 : Constant  Value=0  OutDataTypeStr=Bus: BusGnd
  Demux : Demux
  Demux1 : Demux
  Signal Specification : SignalSpecification  Unit=m
  Signal Specification1 : SignalSpecification  Unit=1
  Vector Concatenate : Concatenate  NumInputs=4
  Vector Concatenate1 : Concatenate  NumInputs=4
  Ground : Outport  VectorParamsAs1DForOutWhenUnconnected=off
  wires:
  Constant4/1 -> Bus Assignment/1
  Vector Concatenate1/1 -> Bus Assignment/3, Bus Assignment/4  "Lambda_mu"
  Vector Concatenate/1 -> Bus Assignment/2  "Z"
  Bus Assignment/1 -> Ground/1
  Signal Specification1/1 -> Demux1/1
  Friction/1 -> Signal Specification1/1
  Demux1/2 -> Vector Concatenate1/2  "mu_FR"
  Demux1/1 -> Vector Concatenate1/1  "mu_FL"
  Demux1/4 -> Vector Concatenate1/4  "mu_RR"
  Demux1/3 -> Vector Concatenate1/3  "mu_RL"
  Demux/2 -> Vector Concatenate/2  "G_FR_z"
  Demux/3 -> Vector Concatenate/3  "G_RL_z"
  Demux/1 -> Vector Concatenate/1  "G_FL_z"
  Demux/4 -> Vector Concatenate/4  "G_RR_z"
  Signal Specification/1 -> Demux/1
  Wheels Elevation/1 -> Signal Specification/1

== system VehDyn14DOF/Input Routing/Vehicle Reference ==
  Bus Assignment : BusAssignment  AssignedSignals=LngRef,LtrRef,XRef,YRef,PhiRef,CurvRef,CurvGradRef
  Constant : Constant  Value=zeros(2,1)  SampleTime=-1
  Constant1 : Constant  Value=0  OutDataTypeStr=Bus: BusVehRef  SampleTime=-1
  Constant{2,4..8} (6 alike) : Constant  Value=0  SampleTime=-1
  Constant3 : Constant  Value=egoVehDyn.VLong0  SampleTime=-1
  Terminator : Terminator
  VehRef : Outport
  wires:
  Bus Assignment/1 -> VehRef/1
  Constant1/1 -> Bus Assignment/1
  Constant8/1 -> Bus Assignment/6  "phiRef"
  Constant/1 -> Terminator/1  "XYPath"
  Constant2/1 -> Bus Assignment/7  "CurvRef"
  Constant7/1 -> Bus Assignment/8  "CurvGradRef"
  Constant4/1 -> Bus Assignment/3  "LtrlRef"
  Constant5/1 -> Bus Assignment/4  "XRef"
  Constant6/1 -> Bus Assignment/5  "YRef"
  Constant3/1 -> Bus Assignment/2  "LngRef"

== system VehDyn14DOF/Passenger Vehicle/Chassis Input ==
  Env : Inport
  Driveline : Inport  Port=2
  Bus Selector : BusSelector  OutputSignals=Wind,Gnd.Z,Gnd.lambda_mux,Gnd.lambda_muy
  Bus Selector4 : BusSelector  OutputSignals=WhlAng,AxlTrq,BrkPrs
  Wind : Outport  VectorParamsAs1DForOutWhenUnconnected=off
  Gnd : Outport  Port=2  VectorParamsAs1DForOutWhenUnconnected=off
  lambda_mux : Outport  Port=3  VectorParamsAs1DForOutWhenUnconnected=off
  lambda_muy : Outport  Port=4  VectorParamsAs1DForOutWhenUnconnected=off
  WhlAng : Outport  Port=5  VectorParamsAs1DForOutWhenUnconnected=off
  AxlTrq : Outport  Port=6  VectorParamsAs1DForOutWhenUnconnected=off
  BrkPrs : Outport  Port=7  VectorParamsAs1DForOutWhenUnconnected=off
  wires:
  Driveline/1 -> Bus Selector4/1
  Bus Selector4/2 -> AxlTrq/1  "<AxlTrq>"
  Bus Selector4/1 -> WhlAng/1  "<WhlAng>"
  Bus Selector4/3 -> BrkPrs/1  "<BrkPrs>"
  Env/1 -> Bus Selector/1
  Bus Selector/1 -> Wind/1  "<Wind>"
  Bus Selector/2 -> Gnd/1  "<Z>"
  Bus Selector/3 -> lambda_mux/1  "<lambda_mux>"
  Bus Selector/4 -> lambda_muy/1  "<lambda_muy>"

== system VehDyn14DOF/Passenger Vehicle/Chassis Output ==
  Veh : Inport
  Wheels : Inport  Port=2
  Out Bus Element4 : Outport  PortName=VehFdbk
  Out Bus Element1 : Outport  Port=2  PortName=WheelsFdbk
  wires:
  Veh/1 -> Out Bus Element4/1
  Wheels/1 -> Out Bus Element1/1

== system VehDyn14DOF/Passenger Vehicle/Chassis and Tires ==
  WindXYZ : Inport  Unit=m/s  PortDimensions=3
  Ground : Inport  Port=2  Unit=m  PortDimensions=4
  FrictionScalingX : Inport  Port=3  Unit=1  PortDimensions=4
  FrictionScalingY : Inport  Port=4  Unit=1  PortDimensions=4
  WhlAng : Inport  Port=5  Unit=rad  PortDimensions=4
  AxlTrq : Inport  Port=6  Unit=N*m  PortDimensions=4
  BrkPrs : Inport  Port=7  PortDimensions=4
  Bus Selector : BusSelector  OutputSignals=InertFrm,BdyFrm  OutputAsBus=on
  Bus Selector1 : BusSelector  OutputSignals=TireFrame,Steering  OutputAsBus=on
  Suspension : Subsystem  Variant=on  VariantControlMode=label  LabelModeActiveChoice=6
      mask Display:
      | switch str2num(get_param(gcb,'ActiveVariant'))
      |     case 1
      |         image('suspdw.png');
      |     case 2
      |         image([imread('suspindmap.png');imread('suspsamap.png')]);
      |     case 3
      |          image([imread('suspmacp.png');imread('suspsacoil.png')]);
      |     case 4
      |          image('suspmacp.png');
      |     case 5
      |          image('suspindmap.png');
      |     case 6
      |          image('suspkandc.png');
      | end
  Vehicle : Subsystem
      mask Display: image('6dofcar.png');
  Wheels and Tires : Subsystem
      mask Display: image('wheel3dof.png')
  Veh : Outport
  Wheels : Outport  Port=2
  wires:
  Wheels and Tires/2(Wheels2Susp) -> Suspension/3(Wheel)
  WhlAng/1 -> Suspension/1(Steering)
  Vehicle/1(VehFdbk) -> Bus Selector/1, Wheels and Tires/1(Veh), Suspension/2(Vehicle)  "Veh"
  Suspension/1(Suspension) -> Wheels and Tires/2(Suspension), Vehicle/1(Suspension)  "Susp"
  Wheels and Tires/1(Wheels) -> Bus Selector1/1  "Wheels"
  Bus Selector/1 -> Veh/1
  WindXYZ/1 -> Vehicle/2(Wind)
  Bus Selector1/1 -> Wheels/1
  FrictionScalingY/1 -> Wheels and Tires/7(FrictionScalingY)
  AxlTrq/1 -> Wheels and Tires/3(Axle Torque)
  BrkPrs/1 -> Wheels and Tires/4(Brake Press)
  Ground/1 -> Wheels and Tires/5(Ground Input)
  FrictionScalingX/1 -> Wheels and Tires/6(FrictionScalingX)

== system VehDyn14DOF/Passenger Vehicle/Driveline Input ==
  Cntrl : Inport
  Driver : Inport  Port=2
  EngTrqCmd : Inport  Port=3
  Wheels : Inport  Port=4
  Bus Selector1 : BusSelector  OutputSignals=steer_cmd
  Bus Selector2 : BusSelector  OutputSignals=TireFrame.Omega
  Bus Selector3 : BusSelector  OutputSignals=Transmission.GearCmd,Brake.BrkPrsCmd,Diff.DiffPrsCmd
  Bus Selector4 : BusSelector  OutputSignals=EngTrq
  Data Type Conversion : DataTypeConversion  SaturateOnIntegerOverflow=off  RndMeth=Floor
  Steer : Outport  VectorParamsAs1DForOutWhenUnconnected=off
  EngTrq : Outport  Port=2  VectorParamsAs1DForOutWhenUnconnected=off
  GearCmd : Outport  Port=3  VectorParamsAs1DForOutWhenUnconnected=off
  BrkPrsCmd : Outport  Port=4  VectorParamsAs1DForOutWhenUnconnected=off
  Omega : Outport  Port=5  VectorParamsAs1DForOutWhenUnconnected=off
  DiffPrsCmd : Outport  Port=6  VectorParamsAs1DForOutWhenUnconnected=off
  wires:
  Cntrl/1 -> Bus Selector3/1
  Bus Selector3/1 -> Data Type Conversion/1  "<GearCmd>"
  Driver/1 -> Bus Selector1/1
  Wheels/1 -> Bus Selector2/1
  Bus Selector2/1 -> Omega/1  "<Omega>"
  Bus Selector3/2 -> BrkPrsCmd/1  "<BrkPrsCmd>"
  EngTrqCmd/1 -> Bus Selector4/1
  Bus Selector1/1 -> Steer/1  "<steer_cmd>"
  Bus Selector4/1 -> EngTrq/1  "<EngTrq>"
  Bus Selector3/3 -> DiffPrsCmd/1  "<DiffPrsCmd>"
  Data Type Conversion/1 -> GearCmd/1

== system VehDyn14DOF/Passenger Vehicle/Driveline Output ==
  WhlAng : Inport
  AxlTrq : Inport  Port=2
  BrkPrs : Inport  Port=3
  EngSpd : Inport  Port=4
  PropShftSpd : Inport  Port=5
  StrWhlTrq : Inport  Port=6
  Gear : Inport  Port=7
  Bus Creator1 : BusCreator  Inputs=6
  Bus Creator2 : BusCreator  Inputs=1
  Driveline : Outport  VectorParamsAs1DForOutWhenUnconnected=off
  Steering : Outport  Port=2  VectorParamsAs1DForOutWhenUnconnected=off
  wires:
  Bus Creator1/1 -> Driveline/1  "Driveline"
  PropShftSpd/1 -> Bus Creator1/5  "PropShftSpd"
  AxlTrq/1 -> Bus Creator1/2  "AxlTrq"
  WhlAng/1 -> Bus Creator1/1  "WhlAng"
  EngSpd/1 -> Bus Creator1/4  "EngSpd"
  BrkPrs/1 -> Bus Creator1/3  "BrkPrs"
  StrWhlTrq/1 -> Bus Creator2/1  "StrWhlTrq"
  Bus Creator2/1 -> Steering/1  "Steering"
  Gear/1 -> Bus Creator1/6  "Gear"
